simulink model "recursive_arx"  (R2019a)
settings: Solver=ode45  StartTime=0.0  StopTime=10.0  RelTol=1e-3
undefined symbols (not defined in the file): den, num, R, S, T
settings Model: Creator=Carlos Henrique  LastModifiedBy=PICHAU
settings DataIOCC: SaveFormat=StructureWithTime  ReturnWorkspaceOutputs=off
settings OptimizationCC: LifeSpan=inf
settings DebuggingCC: SFExecutionAtInitializationDiag=none  ArithmeticOperatorsInVariantConditions=warning
settings HardwareCC: ProdBitPerSizeT=32  ProdBitPerPtrDiffT=32  ProdWordSize=32  ProdHWDeviceType=Specified
settings CodeAppCC: StateflowObjectComments=on

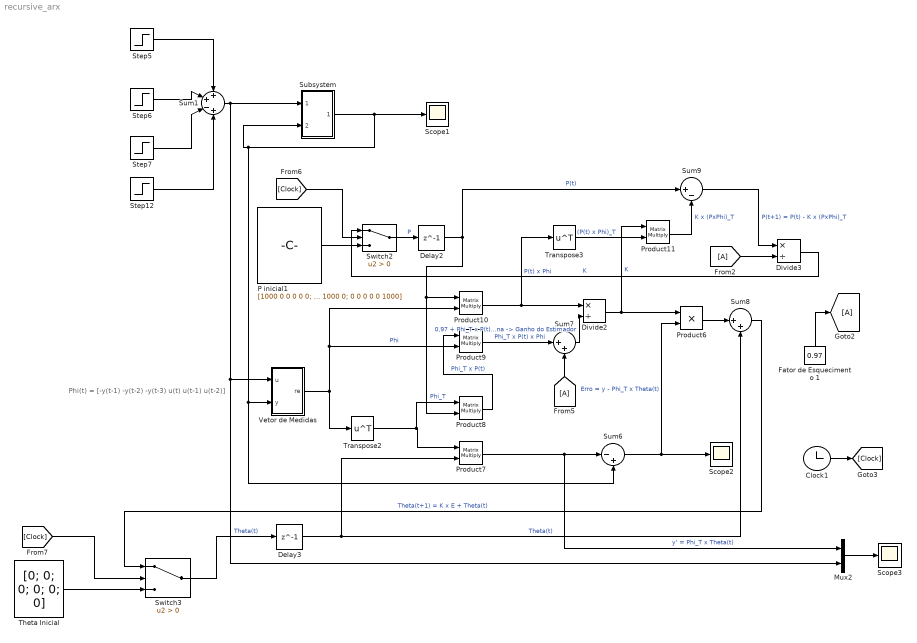
== system recursive_arx ==
  note: Phi(t) = [-y(t-1) -y(t-2) -y(t-3) u(t) u(t-1) u(t-2)]
  Clock1 : Clock
  Delay2 : Delay  DelayLength=1  InitialCondition=0  SampleTime=0.1
  Delay3 : Delay  DelayLength=1  InitialCondition=0  SampleTime=0.1
  Divide2 : Product  Inputs=*/
  Divide3 : Product  Inputs=*/
  Fator de Esquecimento 1 : Constant  Value=0.97
  Mux2 : Mux  Inputs=2
  P inicial1 : Constant  Value=[1000 0 0 0 0 0; 0 1000 0 0 0 0; 0 0 1000 0 0 0; 0 0 0 1000 0 0; 0 0 0 0 1000 0; 0 0 0 0 0 1000]
  Product{7..11} (5 alike) : Product  Multiplication=Matrix(*)
  Product6 : Product
  Scope1 : Scope
  Scope2 : Scope
  Scope3 : Scope
  Step12 : Step  Time=30  SampleTime=0
  Step5 : Step  Time=0  SampleTime=0
  Step6 : Step  Time=10  After=3  SampleTime=0
  Step7 : Step  Time=20  After=2  SampleTime=0
  Subsystem : Subsystem
  Sum1 : Sum  Inputs=++-+
  Sum6 : Sum  Inputs=|-+
  Sum7 : Sum  Inputs=|++
  Sum8 : Sum  Inputs=|++
  Sum9 : Sum  Inputs=|+-
  Switch2 : Switch  Criteria=u2 > Threshold
  Switch3 : Switch  Criteria=u2 > Threshold
  "Theta Inicial " : Constant  Value=[0; 0; 0; 0; 0; 0]
  Transpose2 : Math  Operator=transpose  SaturateOnIntegerOverflow=on
  Transpose3 : Math  Operator=transpose  SaturateOnIntegerOverflow=on
  "Vetor de Medidas " : Subsystem
  wires:
  Step12/1 -> Sum1/4
  Step7/1 -> Sum1/3
  Step6/1 -> Sum1/2
  Step5/1 -> Sum1/1
  Sum1/1 -> Mux2/2, "Vetor de Medidas "/1(u), Subsystem/1(In1)
  Subsystem/1(Out1) -> Subsystem/2(In2), "Vetor de Medidas "/2(y), Sum6/2, Scope1/1
  Mux2/1 -> Scope3/1
  Sum6/1 -> Scope2/1, Product6/2  "Erro = y - Phi_T x Theta(t)"
  Product7/1 -> Mux2/1, Sum6/1  "y' = Phi_T x Theta(t)"
  [A] -> Sum7/2
  Clock1/1 -> [Clock]
  [Clock] -> Switch3/2
  Delay3/1 -> Sum8/2, Product7/2  "Theta(t)"
  Switch3/1 -> Delay3/1  "Theta(t)"
  Product11/1 -> Sum9/2  "K x (PxPhi)_T"
  Delay2/1 -> Product10/1, Product8/2, Sum9/1  "P(t)"
  Sum8/1 -> Switch3/1  "Theta(t+1) = K x E + Theta(t)"
  Transpose2/1 -> Product8/1, Product7/1  "Phi_T"
  [Clock] -> Switch2/2
  "Vetor de Medidas "/1(re) -> Transpose2/1, Product10/2, Product9/2  "Phi"
  Divide2/1 -> Product11/1, Product6/1  "K"
  Sum7/1 -> Divide2/2  "0,97 + Phi_T x P(t) x Phi Vetor Coluna -> Ganho do Estimador"
  Product8/1 -> Product9/1  "Phi_T x P(t)"
  Divide3/1 -> Switch2/1  "K"
  "Theta Inicial "/1 -> Switch3/3
  Product9/1 -> Sum7/1  "Phi_T x P(t) x Phi"
  Transpose3/1 -> Product11/2  "(P(t) x Phi)_T"
  P inicial1/1 -> Switch2/3
  Sum9/1 -> Divide3/1  "P(t+1) = P(t) - K x (PxPhi)_T"
  Product6/1 -> Sum8/1
  [A] -> Divide3/2
  Fator de Esquecimento 1/1 -> [A]
  Product10/1 -> Transpose3/1, Divide2/1  "P(t) x Phi"
  Switch2/1 -> Delay2/1  "P"

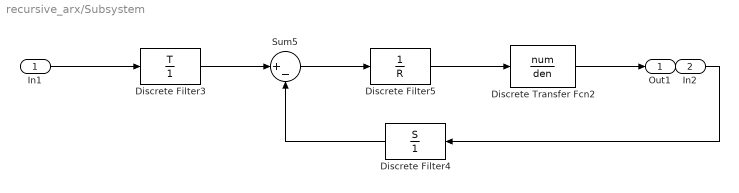
== system recursive_arx/Subsystem ==
  In1 : Inport
  In2 : Inport  Port=2
  Discrete Transfer Fcn2 : DiscreteTransferFcn  Numerator=num  Denominator=den
  Discrete Filter3 : DiscreteFilter  Numerator=T  Denominator=1
  Discrete Filter4 : DiscreteFilter  Numerator=S  Denominator=1
  Discrete Filter5 : DiscreteFilter  Numerator=1  Denominator=R
  Sum5 : Sum  Inputs=|+-
  Out1 : Outport
  wires:
  Discrete Filter5/1 -> Discrete Transfer Fcn2/1
  Discrete Transfer Fcn2/1 -> Out1/1
  Sum5/1 -> Discrete Filter5/1
  In2/1 -> Discrete Filter4/1
  Discrete Filter3/1 -> Sum5/1
  In1/1 -> Discrete Filter3/1
  Discrete Filter4/1 -> Sum5/2

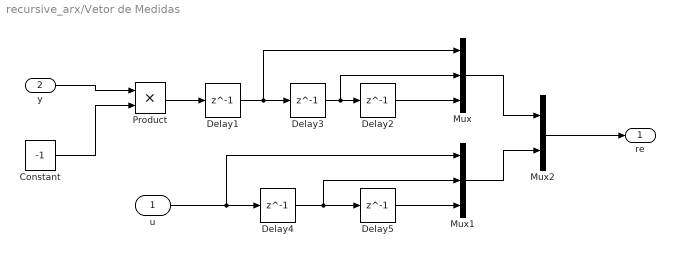
== system recursive_arx/Vetor de Medidas  ==
  u : Inport
  y : Inport  Port=2
  Constant : Constant  Value=-1
  Delay{1..5} (5 alike) : Delay  DelayLength=1  InitialCondition=0  SampleTime=0.1
  Mux : Mux  Inputs=3
  Mux1 : Mux  Inputs=3
  Mux2 : Mux  Inputs=2
  Product : Product
  re : Outport
  wires:
  Delay4/1 -> Mux1/2, Delay5/1
  Delay5/1 -> Mux1/3
  Mux1/1 -> Mux2/2
  Mux/1 -> Mux2/1
  Mux2/1 -> re/1
  u/1 -> Mux1/1, Delay4/1
  Delay2/1 -> Mux/3
  y/1 -> Product/1
  Constant/1 -> Product/2
  Product/1 -> Delay1/1
  Delay3/1 -> Mux/2, Delay2/1
  Delay1/1 -> Mux/1, Delay3/1
